simulink model "GyroSimulation_2016a"  (R2016a)
settings: Solver=ode45  SolverMode=SingleTasking  StartTime=0.0  StopTime=70.0  RelTol=1e-3
InitFcn:
  | InitGyro
undefined symbols (not defined in the file or in its folder): Dr, Du, sigbuilder_block
undefined symbols (not defined in the file): q1dot_0, q2_0, q3_0, sys
libraries: simulink_extras x5, simulink x2, cstblocks x1
settings Model: Creator=jt  LastModifiedBy=Saeed
settings DataIOCC: LimitDataPoints=on  SaveFormat=Array
settings OptimizationCC: BlockReduction=off  BooleanDataType=off
settings DebuggingCC: SaveWithParameterizedLinksMsg=none  UnderspecifiedInitializationDetection=Classic  MergeDetectMultiDrivingBlocksExec=none  SignalResolutionControl=TryResolveAllWithWarning
settings HardwareCC: ProdBitPerPointer=32  ProdLargestAtomicFloat=None  ProdIntDivRoundTo=Undefined  ProdEndianess=Unspecified  ProdWordSize=32  ProdHWDeviceType=32-bit Generic  TargetUnknown=on
settings ModelReferenceCC: PropagateSignalLabelsOutOfModel=off
settings ConfigComp: CovSFcnEnable=off

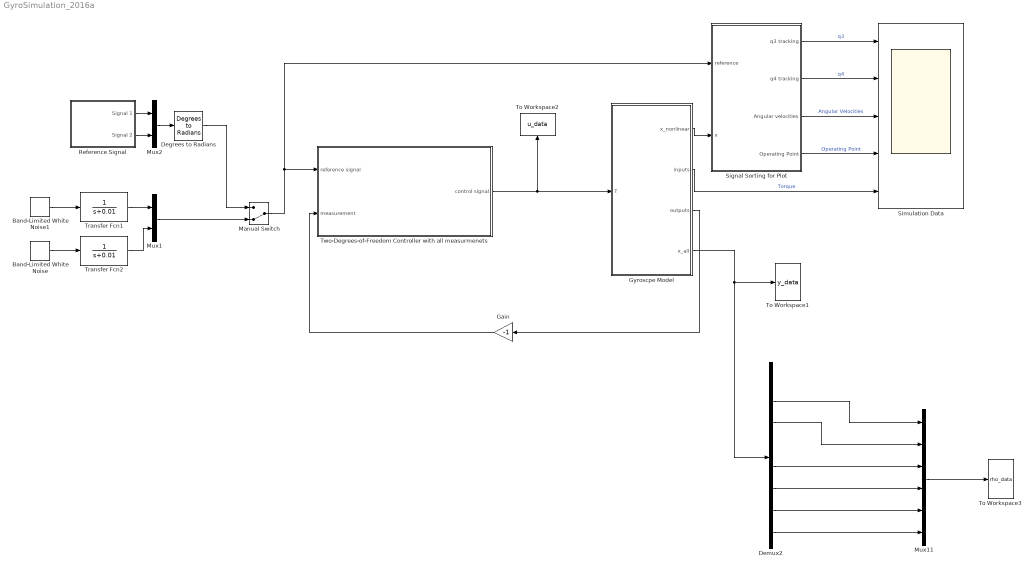
== system GyroSimulation_2016a ==
  Band-Limited White Noise : simulink/Sources/Band-Limited White Noise  Cov=[0.01]  Ts=0.01  seed=[3453]
  Band-Limited White Noise1 : simulink/Sources/Band-Limited White Noise  Cov=[0.01]  Ts=0.01  seed=[23341]
  Degrees to Radians : simulink_extras/Transformations/Degrees to Radians
  Demux2 : Demux  Outputs=8
  Gain : Gain  Gain=-1
  Gyroscpe Model : Subsystem
  Manual Switch : ManualSwitch  CurrentSetting=0
  Mux1 : Mux  Inputs=2
  Mux11 : Mux  Inputs=6
  Mux2 : Mux  Inputs=2
  Reference Signal : Subsystem  Tag=STV Subsys  LoadFcn=sigbuilder_block('load');  StartFcn=sigbuilder_block('start');  StopFcn=sigbuilder_block('stop');  ClipboardFcn=sigbuilder_block('clipboard');  mask(Sigbuilder block){}
      mask help: Sigbuilder GUI
      mask init:
      | if ~strcmp(get_param(bdroot(gcbh),'SimulationStatus'),'stopped') tuvar = sigbuilder_block('maskInit'); end
      settings: CopyFcn=sigbuilder_block('copy');  DeleteFcn=sigbuilder_block('delete');  ModelCloseFcn=sigbuilder_block('modelClose');  PreSaveFcn=sigbuilder_block('preSave');  PauseFcn=sigbuilder_block('pause')  ContinueFcn=sigbuilder_block('continue')  NameChangeFcn=sigbuilder_block('namechange');  OpenFcn=sigbuilder_block('open',[6 0 1428 718.5 ]);  CloseFcn=sigbuilder_block('close');
      mask Display: plot(0, 0, 100, 100,[2, 2, 32, 32, 2], [68, 8, 8, 68, 68],[32, 2], [38, 38], [32, 19, 2],[53, 60, 44], [32, 17, 17, 2],[16, 16, 31, 31]);txt = getActiveGroup(gcbh);text(2, 100, txt,'verticalAlignment', 'top');
  Signal Sorting for Plot : Subsystem
  Simulation Data : Scope  NumInputPorts=5
  To Workspace1 : ToWorkspace  VariableName=y_data  SaveFormat=Timeseries  SampleTime=-1
  To Workspace2 : ToWorkspace  VariableName=u_data  SaveFormat=Timeseries  SampleTime=-1
  To Workspace3 : ToWorkspace  VariableName=rho_data  SaveFormat=Timeseries  SampleTime=-1
  Transfer Fcn1 : TransferFcn  Denominator=[1 0.01]
  Transfer Fcn2 : TransferFcn  Denominator=[1 0.01]
  Two-Degrees-of-Freedom Controller with all measurmenets : Subsystem
  wires:
  Gyroscpe Model/2(inputs) -> Simulation Data/5  "Torque"
  Gyroscpe Model/1(x_nonlinear) -> Signal Sorting for Plot/2(x)
  Mux2/1 -> Degrees to Radians/1
  Reference Signal/1(Signal 1) -> Mux2/1
  Reference Signal/2(Signal 2) -> Mux2/2
  Manual Switch/1 -> Signal Sorting for Plot/1(reference), Two-Degrees-of-Freedom Controller with all measurmenets/1(reference signal)
  Gyroscpe Model/3(outputs) -> Gain/1
  Signal Sorting for Plot/1(q3 tracking) -> Simulation Data/1  "q3"
  Signal Sorting for Plot/2(q4 tracking) -> Simulation Data/2  "q4"
  Signal Sorting for Plot/3(Angular velocities) -> Simulation Data/3  "Angular Velocities"
  Signal Sorting for Plot/4(Operating Point) -> Simulation Data/4  "Operating Point"
  Gain/1 -> Two-Degrees-of-Freedom Controller with all measurmenets/2(measurement)
  Two-Degrees-of-Freedom Controller with all measurmenets/1(control signal) -> Gyroscpe Model/1(T), To Workspace2/1
  Band-Limited White Noise1/1 -> Transfer Fcn1/1
  Band-Limited White Noise/1 -> Transfer Fcn2/1
  Degrees to Radians/1 -> Manual Switch/1
  Mux1/1 -> Manual Switch/2
  Transfer Fcn1/1 -> Mux1/1
  Transfer Fcn2/1 -> Mux1/2
  Gyroscpe Model/4(x_all) -> To Workspace1/1, Demux2/1
  Demux2/2 -> Mux11/1
  Demux2/3 -> Mux11/2
  Demux2/5 -> Mux11/3
  Demux2/6 -> Mux11/4
  Demux2/8 -> Mux11/6
  Demux2/7 -> Mux11/5
  Mux11/1 -> To Workspace3/1

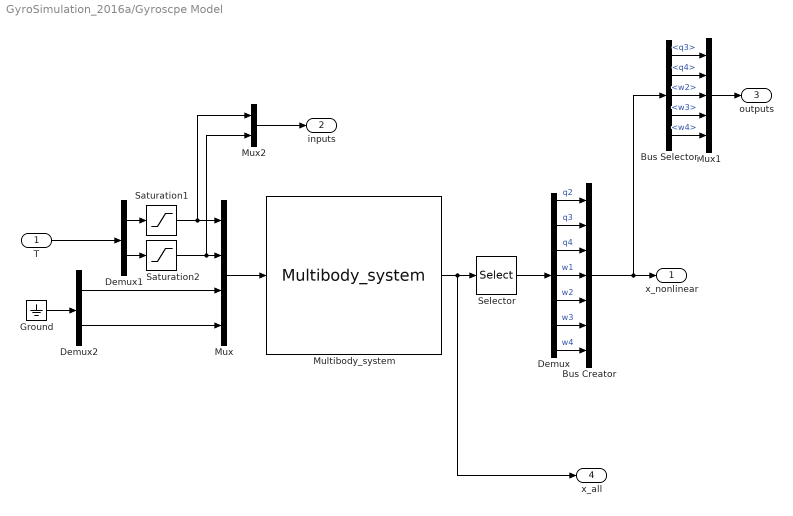
== system GyroSimulation_2016a/Gyroscpe Model ==
  T : Inport
  Bus Creator : BusCreator  Inputs=7
  Bus Selector : BusSelector  OutputSignals=q3,q4,w2,w3,w4
  Demux : Demux  Outputs=7
  Demux1 : Demux  Outputs=2
  Demux2 : Demux  Outputs=2
  Ground : Ground
  Multibody_system : S-Function  FunctionName=Multibody_system  Parameters=paraStruct, initY, initDy  SFunctionDeploymentMode=off  EnableBusSupport=off  mask(Neweul-M2 nonlinear model){paraStruct=sys.parameters.data, initY=[0 q2_0 q3_0 0]';, initDy=[q1dot_0 0 0 0]';}
      mask prompts: paraStruct "Neweul-M2 Parameter Structure"; initY "Initial coordinates"; initDy "Initial velocities"
      mask help:
      | State-state representation of a multibody system
      | created with Neueul-MÂ².
      |
      | In order to run a simulation in Simulink you have to provide
      | the following input parameters:
      |   * Neweul-M2 Parameter Structure (sys.parameters.data)
      |     ... Structure containing all user-defined parameters
      |   * Initial coordinates (zeros(sys.counters.genCoord,1))
      |     ... Initial values for the generalized coordinates
      |   * Initial velocities (zeros(sys.dof,1))
      |     ... Initial values for the generalized velocities
      |
      | Neweul-MÂ²
      | Multibody systems based on symbolic Newton-Euler-Equations
      | Copyright (c) ITM University of Stuttgart, www.itm.uni-stuttgart.de
      mask Display:
      | port_label('output',1,'states [8x1]');
      | port_label('input',1,'control [4x1]');
  Mux : Mux
  Mux1 : Mux  Inputs=5
  Mux2 : Mux  Inputs=2
  Saturation1 : Saturate  UpperLimit=0.666  LowerLimit=-0.666
  Saturation2 : Saturate  UpperLimit=2.44  LowerLimit=-2.44
  Selector : Selector  IndexOptions=Index vector (dialog)  Indices=2:8  OutputSizes=1
  x_nonlinear : Outport
  inputs : Outport  Port=2
  outputs : Outport  Port=3
  x_all : Outport  Port=4
  wires:
  Multibody_system/1 -> x_all/1, Selector/1
  Demux/6 -> Bus Creator/6  "w3"
  Demux/3 -> Bus Creator/3  "q4"
  Demux/1 -> Bus Creator/1  "q2"
  Demux/2 -> Bus Creator/2  "q3"
  Demux/7 -> Bus Creator/7  "w4"
  Selector/1 -> Demux/1
  Bus Creator/1 -> Bus Selector/1, x_nonlinear/1
  Mux/1 -> Multibody_system/1
  Demux2/2 -> Mux/4
  Demux2/1 -> Mux/3
  Demux1/2 -> Saturation2/1
  Demux/5 -> Bus Creator/5  "w2"
  Demux/4 -> Bus Creator/4  "w1"
  Mux2/1 -> inputs/1
  Saturation2/1 -> Mux2/2, Mux/2
  Saturation1/1 -> Mux2/1, Mux/1
  Mux1/1 -> outputs/1
  Demux1/1 -> Saturation1/1
  T/1 -> Demux1/1
  Ground/1 -> Demux2/1
  Bus Selector/1 -> Mux1/1  "<q3>"
  Bus Selector/2 -> Mux1/2  "<q4>"
  Bus Selector/3 -> Mux1/3  "<w2>"
  Bus Selector/4 -> Mux1/4  "<w3>"
  Bus Selector/5 -> Mux1/5  "<w4>"

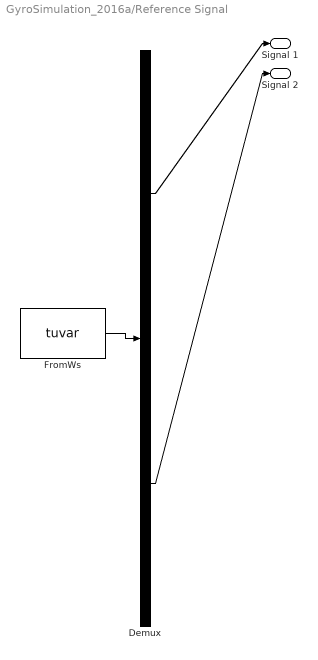
== system GyroSimulation_2016a/Reference Signal ==
  Demux : Demux  Tag=STV Demux  Outputs=2
  FromWs : FromWorkspace  Tag=STV FromWs  VariableName=tuvar  SampleTime=0
      SigBuilderData=|
      | common.afterFinalStr = 'Extrapolate'
      | common.sampleTime = 0
      | dataSet.timeRange = [0 70]
      | dataSet.name = 'Group 1'
      | sbobj.Groups.Name = 'Group 1'
      | sbobj.Groups.Signals(1).Name = 'Signal 1'
      | sbobj.Groups.Signals(1).XData = [0 22 22 28 28 34 34 40 40 46 46 52 52 58 58 64 64 70]
      | sbobj.Groups.Signals(1).YData = [0 0 -5 -5 0 0 5 5 0 0 -5 -5 0 0 5 5 0 0]
      | sbobj.Groups.Signals(2).Name = 'Signal 2'
      | sbobj.Groups.Signals(2).XData = [0 25 25 37 37 49 49 61 61 70]
      | sbobj.Groups.Signals(2).YData = [0 0 -40 -40 0 -0.2 40 40 -0.2 -0.2]
      | sbobj.Groups.TimeRange = [0 70]
  Signal 1 : Outport  Tag=STV Outport
  Signal 2 : Outport  Tag=STV Outport  Port=2
  wires:
  FromWs/1 -> Demux/1
  Demux/1 -> Signal 1/1
  Demux/2 -> Signal 2/1

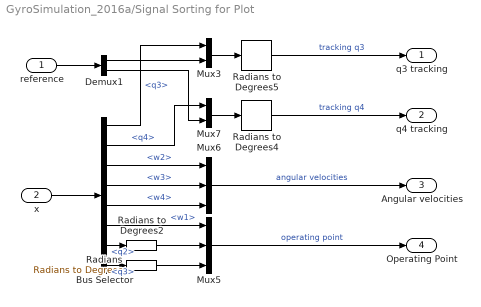
== system GyroSimulation_2016a/Signal Sorting for Plot ==
  reference : Inport
  x : Inport  Port=2
  Bus Selector : BusSelector  OutputSignals=q3,q4,w2,w3,w4,w1,q2,q3
  Demux1 : Demux  Outputs=2
  Mux3 : Mux  Inputs=2
  Mux5 : Mux  Inputs=3
  Mux6 : Mux  Inputs=3
  Mux7 : Mux  Inputs=2
  "Radians " : simulink_extras/Transformations/Radians to Degrees
  Radians to Degrees2 : simulink_extras/Transformations/Radians to Degrees
  Radians to Degrees4 : simulink_extras/Transformations/Radians to Degrees
  Radians to Degrees5 : simulink_extras/Transformations/Radians to Degrees
  q3 tracking : Outport
  q4 tracking : Outport  Port=2
  Angular velocities : Outport  Port=3
  Operating Point : Outport  Port=4
  wires:
  Bus Selector/3 -> Mux6/1  "<w2>"
  Bus Selector/2 -> Mux7/1  "<q4>"
  Radians to Degrees4/1 -> q4 tracking/1  "tracking q4"
  Mux3/1 -> Radians to Degrees5/1
  Radians to Degrees5/1 -> q3 tracking/1  "tracking q3"
  Mux7/1 -> Radians to Degrees4/1
  Demux1/1 -> Mux3/2
  Demux1/2 -> Mux7/2
  Bus Selector/1 -> Mux3/1  "<q3>"
  Mux6/1 -> Angular velocities/1  "angular velocities"
  Bus Selector/5 -> Mux6/3  "<w4>"
  Bus Selector/4 -> Mux6/2  "<w3>"
  Mux5/1 -> Operating Point/1  "operating point"
  Bus Selector/6 -> Mux5/1  "<w1>"
  Bus Selector/7 -> Radians to Degrees2/1  "<q2>"
  Bus Selector/8 -> "Radians "/1  "<q3>"
  "Radians "/1 -> Mux5/3
  Radians to Degrees2/1 -> Mux5/2
  reference/1 -> Demux1/1
  x/1 -> Bus Selector/1

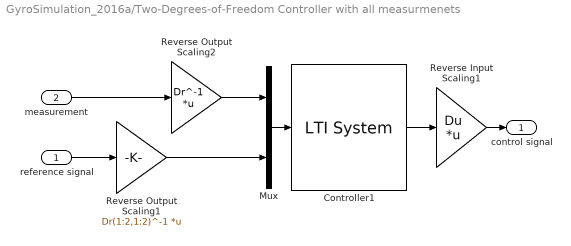
== system GyroSimulation_2016a/Two-Degrees-of-Freedom Controller with all measurmenets ==
  reference signal : Inport
  measurement : Inport  Port=2
  Controller1 : cstblocks/LTI System  sys=K3  IC=[]
  Mux : Mux  Inputs=2
  Reverse Input Scaling1 : Gain  Gain=Du  Multiplication=Matrix(K*u)
  Reverse Output Scaling1 : Gain  Gain=Dr(1:2,1:2)^-1  Multiplication=Matrix(K*u)
  Reverse Output Scaling2 : Gain  Gain=Dr^-1  Multiplication=Matrix(K*u)
  control signal : Outport
  wires:
  Reverse Output Scaling1/1 -> Mux/2
  Reverse Output Scaling2/1 -> Mux/1
  measurement/1 -> Reverse Output Scaling2/1
  Mux/1 -> Controller1/1
  Controller1/1 -> Reverse Input Scaling1/1
  Reverse Input Scaling1/1 -> control signal/1
  reference signal/1 -> Reverse Output Scaling1/1
